simulink model "DMC_Model"  (R2022b)
settings: Solver=FixedStepAuto  StartTime=0.0  StopTime=100.0  FixedStep=0.01  RelTol=1e-3
undefined symbols (not defined in the file): Ks, Ts
settings Model: Creator=artur  LastModifiedBy=artur

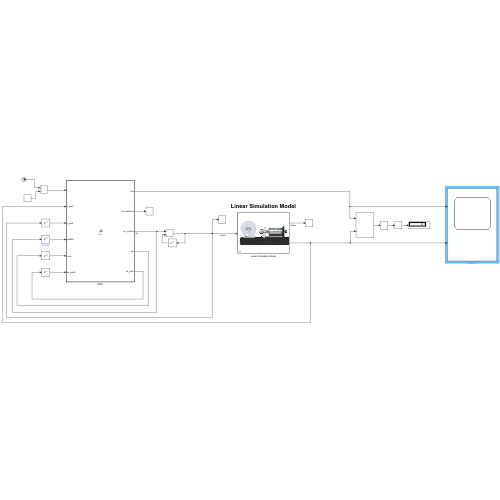
[thumbnail: Simulink's stored preview of the top-level diagram]
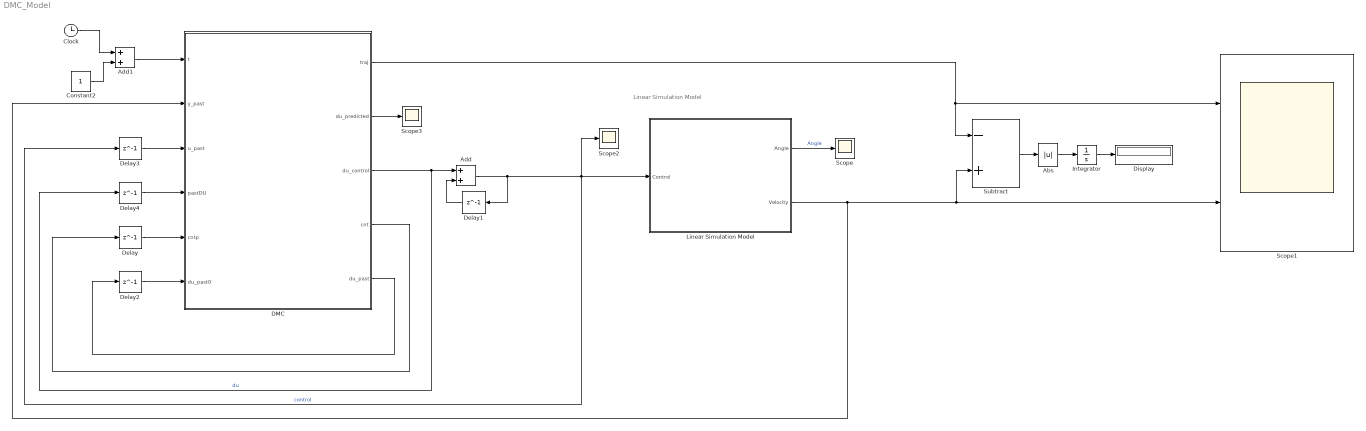
== system DMC_Model ==
  note: Linear Simulation Model
  Abs : Abs  SaturateOnIntegerOverflow=off
  Add : Sum
  Add1 : Sum
  Clock : Clock
  Constant2 : Constant
  DMC : MATLAB Function  TreatAsAtomicUnit=on
  Delay : Delay  DelayLength=1  InitialCondition=1
  Delay1 : Delay  DelayLength=1  InitialCondition=0
  Delay2 : Delay  DelayLength=1  InitialCondition=zeros(1,100-1)
  Delay3 : Delay  DelayLength=1  InitialCondition=0
  Delay4 : Delay  DelayLength=1  InitialCondition=0
  Display : Display
  Integrator : Integrator
  Linear Simulation Model : Subsystem  mask{x0=[0 0]}
      mask prompts: x0 "Initial conditions [angle vel]"
      mask Display: image(imread('Servo_m.JPG'))
  Scope : Scope
  Scope1 : Scope  NumInputPorts=2
  Scope2 : Scope
  Scope3 : Scope
  Subtract : Sum  Inputs=-+
  wires:
  Linear Simulation Model/1(Angle) -> Scope/1  "Angle"
  DMC/4(cnt) -> Delay/1
  Delay/1 -> DMC/5(cntp)
  Delay1/1 -> Add/2
  DMC/3(du_control) -> Add/1, Delay4/1  "du"
  DMC/2(du_predicted) -> Scope3/1
  Add1/1 -> DMC/1(t)
  Delay3/1 -> DMC/3(u_past)
  Delay4/1 -> DMC/4(pastDU)
  DMC/1(traj) -> Scope1/1, Subtract/1
  Integrator/1 -> Display/1
  Abs/1 -> Integrator/1
  Subtract/1 -> Abs/1
  DMC/5(du_past) -> Delay2/1
  Delay2/1 -> DMC/6(du_past0)
  Add/1 -> Delay1/1, Linear Simulation Model/1(Control), Scope2/1, Delay3/1  "control"
  Linear Simulation Model/2(Velocity) -> DMC/2(y_past), Scope1/2, Subtract/2
  Constant2/1 -> Add1/2
  Clock/1 -> Add1/1

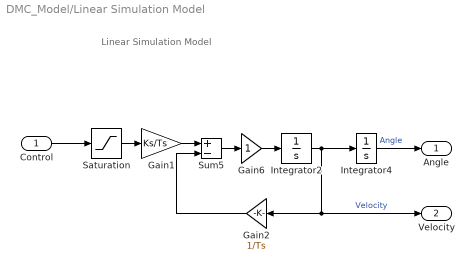
== system DMC_Model/Linear Simulation Model ==
  note: Linear Simulation Model
  Control : Inport
  Gain1 : Gain  Gain=Ks/Ts  SaturateOnIntegerOverflow=on  OutDataTypeStr=Inherit: Same as input  ParamDataTypeStr=Inherit: Same as input
  Gain2 : Gain  Gain=1/Ts  SaturateOnIntegerOverflow=on  OutDataTypeStr=Inherit: Same as input  ParamDataTypeStr=Inherit: Same as input
  Gain6 : Gain  SaturateOnIntegerOverflow=on  OutDataTypeStr=Inherit: Same as input  ParamDataTypeStr=Inherit: Same as input
  Integrator2 : Integrator  InitialCondition=x0(2)
  Integrator4 : Integrator  InitialCondition=x0(1)
  Saturation : Saturate  UpperLimit=1  LowerLimit=-1
  Sum5 : Sum  Inputs=+-  InputSameDT=on  SaturateOnIntegerOverflow=on  OutDataTypeStr=Inherit: Same as first input
  Angle : Outport  InitialOutput=0  VectorParamsAs1DForOutWhenUnconnected=off
  Velocity : Outport  Port=2  InitialOutput=0  VectorParamsAs1DForOutWhenUnconnected=off
  wires:
  Sum5/1 -> Gain6/1
  Gain2/1 -> Sum5/2
  Integrator2/1 -> Integrator4/1, Velocity/1, Gain2/1  "Velocity"
  Integrator4/1 -> Angle/1  "Angle"
  Gain6/1 -> Integrator2/1
  Control/1 -> Saturation/1
  Saturation/1 -> Gain1/1
  Gain1/1 -> Sum5/1

== matlab function DMC_Model/DMC ==
  data: traj output; du_predicted output; t input; y_past input; u_past input; pastDU input; du_control output; cntp input; cnt output; du_past0 input; du_past output
function [traj,du_predicted, du_control,cnt,du_past] = fcn(t,y_past,u_past,pastDU,cntp,du_past0)

cnt = cntp;
    
%Parametry
    ny = 60; %HORYZONT PREDYKCJI
    nu = 20; %HORYZONT STEROWANIA
    lambda = 10;
    D = 100;
    gi = [0	21.4057831151102	40.4617839185735	57.4259456438815	72.5278962583095	85.9720567216218	97.9404080411269	108.594954578115	118.079916949152	126.523684205473	134.040551715317	140.732268273259	146.689413378344	151.992623323918	156.713682695600	160.916496051981	164.657952940772	167.988697959328	170.953816283119	173.593443941528	175.943311101677	178.035225714239	179.897504067869	181.555354080279	183.031216514213	184.345068737025	185.514695135598	186.555927846921	187.482861062907	188.308041810258	189.042639787822	189.696598560338	190.278770155157	190.797034883851	191.258408010603	191.669134711271	192.034774608482	192.360277027037	192.650047988285	192.908009850304	193.137654401192	193.342090124133	193.524084274016	193.686100335178	193.830331367282	193.958729690710	194.073033313299	194.174789456122	194.265375496771	194.346017613628	194.417807383494	194.481716557238	194.538610213484	194.589258468364	194.634346899865	194.674485827849	194.710218575387	194.742028823213	194.770347156855	194.795556895071	194.817999278474	194.837978088585	194.855763759845	194.871597040225	194.885692250011	194.898240182855	194.909410688371	194.919354971229	194.928207637871	194.936088518553	194.943104289376	194.949349916257	194.954909940397	194.959859622636	194.964265962185	194.968188603535	194.971680643808	194.974789351483	194.977556806223	194.980020468472	194.982213686516	194.984166147895	194.985904281249	194.987451614061	194.988829091127	194.990055358063	194.991147013696	194.992118834746	194.992983975844	194.993754147595	194.994439775092	194.995050139033	194.995593501342	194.996077217007	194.996507833632	194.996891180073	194.997232445330	194.997536248791	194.997806702761	194.998047468120	194.998261803884	194.998452611315	194.998622473195	194.998773688785	194.998908304948	194.999028143858	194.999134827663	194.999229800439	194.999314347745	194.999389614020	194.999456618070	194.999516266869	194.999569367825	194.999616639717	194.999658722420	194.999696185568	194.999729536265	194.999759225947	194.999785656497	194.999809185679	194.999830131986	194.999848778950	194.999865378975	194.999880156762	194.999893312344	194.999905023794	194.999915449641	194.999924731008	194.999932993530	194.999940349047	194.999946897126	194.999952726401	194.999957915778	194.999962535499	194.999966648099	194.999970309246	194.999973568496	194.999976469968	194.999979052936	194.999981352363	194.999983399375	194.999985221679	194.999986843944	194.999988288127	194.999989573777	194.999990718297	194.999991737180	194.999992644217	194.999993451685	194.999994170515	194.999994810436	194.999995380111	194.999995887252	194.999996338721	194.999996740632	194.999997098423	194.999997416939	194.999997700490	194.999997952914	194.999998177630	194.999998377677	194.999998555765	194.999998714303	194.999998855438	194.999998981081	194.999999092931	194.999999192503	194.999999281144	194.999999360055	194.999999430304	194.999999492842	194.999999548514	194.999999598075	194.999999642196	194.999999681473	194.999999716439	194.999999747566	194.999999775277	194.999999799945	194.999999821906	194.999999841456	194.999999858860	194.999999874353	194.999999888146	194.999999900424	194.999999911355	194.999999921086	194.999999929749	194.999999937460	194.999999944326	194.999999950437	194.999999955878	194.999999960721	194.999999965033	194.999999968871	194.999999972289	194.999999975330	194.999999978039	194.999999980449	194.999999982595	194.999999984506	194.999999986207	194.999999987721	194.999999989069	194.999999990269	194.999999991337	194.999999992288	194.999999993135	194.999999993888	194.999999994559	194.999999995156	194.999999995688	194.999999996161	194.999999996583	194.999999996958	194.999999997292	194.999999997589	194.999999997854	194.999999998089	194.999999998299	194.999999998486	194.999999998652	194.999999998800	194.999999998932	194.999999999049	194.999999999153	194.999999999246	194.999999999329	194.999999999403	194.999999999468	194.999999999527	194.999999999579	194.999999999625	194.999999999666	194.999999999703	194.999999999735	194.999999999764	194.999999999790	194.999999999813	194.999999999834	194.999999999852	194.999999999868	194.999999999883	194.999999999896	194.999999999907	194.999999999917	194.999999999926	194.999999999934	194.999999999942	194.999999999948	194.999999999954	194.999999999959	194.999999999963	194.999999999967	194.999999999971	194.999999999974	194.999999999977	194.999999999980	194.999999999982	194.999999999984	194.999999999986	194.999999999987	194.999999999989	194.999999999990	194.999999999991	194.999999999992	194.999999999993	194.999999999994	194.999999999994	194.999999999995	194.999999999995	194.999999999996	194.999999999996	194.999999999997	194.999999999997	194.999999999997	194.999999999998	194.999999999998	194.999999999998	194.999999999998	194.999999999999	194.999999999999	194.999999999999	194.999999999999	194.999999999999	194.999999999999	194.999999999999	194.999999999999	194.999999999999	195.000000000000	195.000000000000	195.000000000000	195.000000000000	195.000000000000	195.000000000000	195.000000000000	195.000000000000	195.000000000000	195.000000000000	195.000000000000	195.000000000000	195.000000000000	195.000000000000	195.000000000000	195.000000000000	195.000000000000	195.000000000000	195.000000000000	195.000000000000	195.000000000000	195.000000000000	195.000000000000	195.000000000000	195.000000000000	195.000000000000	195.000000000000	195.000000000000	195.000000000000	195.000000000000	195.000000000000	195.000000000000	195.000000000000	195.000000000000	195.000000000000	195.000000000000	195.000000000000	195.000000000000	195.000000000000	195.000000000000	195.000000000000	195.000000000000	195.000000000000	195.000000000000	195.000000000000	195.000000000000	195.000000000000	195.000000000000	195.000000000000	195.000000000000	195.000000000000	195.000000000000	195.000000000000	195.000000000000	195.000000000000	195.000000000000	195.000000000000	195.000000000000	195.000000000000	195.000000000000	195.000000000000	195.000000000000	195.000000000000	195.000000000000	195.000000000000	195.000000000000	195.000000000000	195.000000000000	195.000000000000	195.000000000000	195.000000000000	195.000000000000	195.000000000000	195.000000000000	195.000000000000	195.000000000000	195.000000000000	195.000000000000	195.000000000000	195.000000000000	195.000000000000	195.000000000000	195.000000000000	195.000000000000	195.000000000000	195.000000000000	195.000000000000	195.000000000000	195.000000000000	195.000000000000	195.000000000000	195.000000000000	195.000000000000	195.000000000000	195.000000000000	195.000000000000	195.000000000000	195.000000000000	195.000000000000	195.000000000000	195.000000000000	195.000000000000	195.000000000000	195.000000000000	195.000000000000	195.000000000000	195.000000000000	195.000000000000	195.000000000000	195.000000000000	195.000000000000	195.000000000000	195.000000000000	195.000000000000	195.000000000000	195.000000000000	195.000000000000	195.000000000000	195.000000000000	195.000000000000	195.000000000000	195.000000000000	195.000000000000	195.000000000000	195.000000000000	195.000000000000	195.000000000000	195.000000000000	195.000000000000	195.000000000000	195.000000000000	195.000000000000	195.000000000000	195.000000000000	195.000000000000	195.000000000000	195.000000000000	195.000000000000	195.000000000000	195.000000000000	195.000000000000	195.000000000000	195.000000000000	195.000000000000	195.000000000000	195.000000000000	195.000000000000	195.000000000000	195.000000000000	195.000000000000	195.000000000000	195.000000000000	195.000000000000	195.000000000000	195.000000000000	195.000000000000	195.000000000000	195.000000000000	195.000000000000	195.000000000000	195.000000000000	195.000000000000	195.000000000000	195.000000000000	195.000000000000	195.000000000000	195.000000000000	195.000000000000	195.000000000000	195.000000000000	195.000000000000	195.000000000000	195.000000000000	195.000000000000	195.000000000000	195.000000000000	195.000000000000	195.000000000000	195.000000000000	195.000000000000	195.000000000000	195.000000000000	195.000000000000	195.000000000000	195.000000000000	195.000000000000	195.000000000000	195.000000000000	195.000000000000	195.000000000000	195.000000000000	195.000000000000	195.000000000000	195.000000000000	195.000000000000	195.000000000000	195.000000000000	195.000000000000	195.000000000000	195.000000000000	195.000000000000	195.000000000000	195.000000000000	195.000000000000	195.000000000000	195.000000000000	195.000000000000	195.000000000000	195.000000000000	195.000000000000	195.000000000000	195.000000000000];
    ograniczenie_wyjscia = false;
    
%Wektor przeszłych du
for i = 1:D-2
    du_past0(D-i) = du_past0(D-1-i);
end

du_past0(1) = pastDU;
du_past = du_past0;


% %Ustawienie ograniczeń dla optymalizatora 
    du_max = 1;
    du_min = -1;
    u_max = 1;
    u_min = -1;
    y_max = 42;
    y_min = -42;

%Trajektoria referencyjna, stała
Ts = 0.1; sim_time = 100; ref = 100;

traj_ub = ref*ones(1/Ts*sim_time/2,1);

traj_lb = -ref*ones(1/Ts*sim_time/2,1);

trajektoria = [traj_ub;traj_lb;traj_lb;-ref*ones(ny,1)];

ref = trajektoria(fix(t/Ts):ny+fix(t/Ts) - 1, 1);

traj = ref(1);

    
%Wyznaczenie macierzy predykcji
    
    [H,P] = dmc_predmat(ny,nu,D,gi);
    Q = ones(ny,1);
    
%Prawo sterowania dla algorytmu z ograniczeniami
    S = H'*H + eye(nu)*lambda;
    S = (S + S')/2;
    f = H'*Q * y_past + H'*P * du_past - H' * ref;

%OGRANICZENIA
    if ograniczenie_wyjscia == true
        %OGRANICZENIA Z Y
        [C,dd,du,ddu,dy] = mpc_ograniczenia(du_max,du_min,u_max,u_min,y_max,y_min,nu,H,P,Q,D-1,1);
        dt = dd + du * u_past + ddu * du_past + dy*y_past;
    else
        %OGRANICZENIA BEZ Y
        [C, dd,du] = mpc_ograniczenia_bez_y(du_max,du_min,u_max,u_min,nu);
        dt = dd + du * u_past;
    end

    opts = optimoptions('quadprog','Algorithm','active-set');

    x0 = 1*eye(nu,1);

    du_predicted = quadprog(S,f,C,dt,[],[],[],[],x0,opts);

    du_control = du_predicted(1);

%Prawo sterowania dla algorytmu bez ograniczeń
% Pr = ( inv(H'*H+lambda*eye(nu)) ) * H';
% Nk = Pr*Q;
% Dk = Pr*P;
% 
% du_predicted = Pr * ref - Dk * du_past - Nk*y_past;
% du_control = du_predicted(1);

%Alternatywne prawo sterowania
% G = H;
% w = ref;
% f = Q *y_past + P * du_past;
% 
% du_predicted = inv(G' * G + lambda*eye(nu) ) * G' * (w - f);
% du_control = du_predicted(1);
